simulink model "propulsion"  (R2025b)
settings: Solver=VariableStepAuto  StartTime=0.0  StopTime=10.0  RelTol=1e-3
undefined symbols (not defined in the file or in its folder): DiscIntNeverNeededParam
settings Model: Creator=taeta  LastModifiedBy=taeta

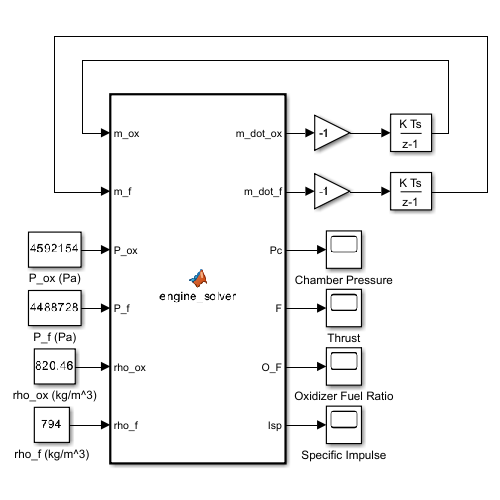
[thumbnail: Simulink's stored preview of the top-level diagram]
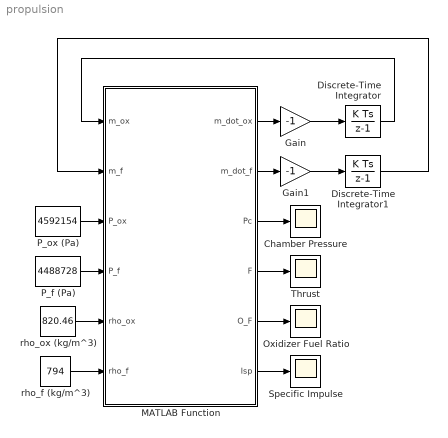
== system propulsion ==
  Chamber Pressure : Scope
      settings: ActiveDisplayYMinimum=-1  ActiveDisplayYMaximum=1
  Discrete-Time Integrator : DiscreteIntegrator  InitialCondition=33.8916  SampleTime=-1  ICPrevOutput=DiscIntNeverNeededParam  ICPrevScaledInput=DiscIntNeverNeededParam
  Discrete-Time Integrator1 : DiscreteIntegrator  InitialCondition=9.678  SampleTime=-1  ICPrevOutput=DiscIntNeverNeededParam  ICPrevScaledInput=DiscIntNeverNeededParam
  Gain : Gain  Gain=-1
  Gain1 : Gain  Gain=-1
  MATLAB Function : MATLAB Function  TreatAsAtomicUnit=on
  Oxidizer Fuel Ratio : Scope
      settings: ActiveDisplayYMinimum=-1  ActiveDisplayYMaximum=1  DataLoggingVariableName=ScopeData2
  P_f (Pa) : Constant  Value=4488728
  P_ox (Pa) : Constant  Value=4592154
  Specific Impulse : Scope
      settings: ActiveDisplayYMinimum=-1  ActiveDisplayYMaximum=1  DataLoggingVariableName=ScopeData3
  Thrust : Scope
      settings: ActiveDisplayYMinimum=-1  ActiveDisplayYMaximum=1
  rho_f (kg/m^3) : Constant  Value=794
  rho_ox (kg/m^3) : Constant  Value=820.46
  wires:
  MATLAB Function/1(m_dot_ox) -> Gain/1
  MATLAB Function/2(m_dot_f) -> Gain1/1
  Discrete-Time Integrator/1 -> MATLAB Function/1(m_ox)
  Discrete-Time Integrator1/1 -> MATLAB Function/2(m_f)
  Gain/1 -> Discrete-Time Integrator/1
  Gain1/1 -> Discrete-Time Integrator1/1
  rho_f (kg/m^3)/1 -> MATLAB Function/6(rho_f)
  rho_ox (kg/m^3)/1 -> MATLAB Function/5(rho_ox)
  P_ox (Pa)/1 -> MATLAB Function/3(P_ox)
  P_f (Pa)/1 -> MATLAB Function/4(P_f)
  MATLAB Function/6(Isp) -> Specific Impulse/1
  MATLAB Function/5(O_F) -> Oxidizer Fuel Ratio/1
  MATLAB Function/4(F) -> Thrust/1
  MATLAB Function/3(Pc) -> Chamber Pressure/1

== matlab function propulsion/MATLAB Function ==
  data: m_ox input; m_dot_ox output; m_f input; P_ox input; P_f input; rho_ox input; rho_f input; m_dot_f output; Pc output; F output; O_F output; Isp output
function [m_dot_ox, m_dot_f, Pc, F, O_F, Isp] = engine_solver(m_ox, m_f, P_ox, P_f, rho_ox, rho_f)

    % output dimensions for simulink (everything equals 0 at first)
    m_dot_ox = 0;
    m_dot_f = 0;
    Pc = 0;
    F = 0;
    O_F = 0;
    Isp = 0;

    % constants
    g0 = 9.81; % m/s^2
    c_star = 2639.4; % m/s
    A_t = 7.85398e-5; % m^2
    A_e = 1.8816e-3; % m^2
    C_f = A_e / A_t; % thrust coefficient

    % initial guesses [m_dot_ox (kg/s); m_dot_f (kg/s); Pc (Pa)]
    x0 = [1.66337; 0.478249; 435.113 * 6894.76];

    % optimization for simulink or else it wont work
    options = optimoptions('fsolve', ...
        'Algorithm', 'levenberg-marquardt', ...
        'Display', 'off', ...
        'FunctionTolerance', 1e-6);

    % solve non-linear residual system
    [x_sol, ~, exitflag] = fsolve(@(x) engine_residuals(x, P_ox, P_f, rho_ox, rho_f, A_t, c_star), x0, options);

    if exitflag <= 0
        x_sol = x0; % so if solver fails to converge it like fixes itself basiaclly
    end

    % gets the solved state values
    m_dot_ox = abs(x_sol(1));
    m_dot_f = abs(x_sol(2));
    Pc = abs(x_sol(3));

    % engine performance outputs
    m_dot_tot = m_dot_ox + m_dot_f;
    F = C_f * Pc * A_t;
    O_F = m_dot_ox / max(m_dot_f, 1e-6);
    Isp = F / (max(m_dot_tot, 1e-6) * g0);
end

function R = engine_residuals(x, P_ox, P_f, rho_ox, rho_f, A_t, c_star)
    m_dot_ox_guess = abs(x(1));
    m_dot_f_guess = abs(x(2));
    Pc_guess = abs(x(3));

    % line losses using oxidizer and fuel constants
    dp_ox = calculate_line_loss_ox(m_dot_ox_guess, rho_ox);
    dp_f = calculate_line_loss_f(m_dot_f_guess, rho_f);

    % residual equations (assuming we want R=0)
    R_ox = P_ox - dp_ox - Pc_guess;
    R_f = P_f - dp_f - Pc_guess;
    R_c = (m_dot_ox_guess + m_dot_f_guess) - (Pc_guess * A_t / c_star);

    R = [R_ox; R_f; R_c];

    % this is so NaN/inf doesnt happen to fsolve
    if any(~isfinite(R))
        R = [1e6; 1e6; 1e6];
    end
end

function dp = calculate_line_loss_ox(m_dot, rho)
    % oxidizer line parameters
    g0 = 9.81;
    rho_safe = max(rho, 1e-3);
    
    f = 0.04; % friction factor
    D = 0.0535088; % pipe diameter (m)
    L = 0.762; % pipe length (m)
    k = 10; % minor loss coefficient
    Cv = 9; % valve flow coefficient
    A_inj = 2.20893e-5; % injector area (m^2)
    dz = 0.9144; % elevation change (m)
    
    % velocity and dynamic pressur
    A_pipe = (pi / 4) * D^2;
    v = m_dot / (rho_safe * A_pipe);
    q = 0.5 * rho_safe * (v^2);

    % individual pressure loss terms
    dp_pipe = f * (L / D) * q; % pipe loss
    dp_k = k * q; % minor loss
    
    % valve loss: i made it so that it converts m_dot to GPM for Cv equation
    SG = rho_safe / 1000; % specific gravity
    Q_gpm = (m_dot / rho_safe) * 15850.32; % m^3/s to GPM
    dp_v = SG * (Q_gpm / Cv)^2 * 6894.76; % converted psi to Pa
    
    dp_inj = 0.5 * (m_dot / A_inj)^2 / rho_safe; % injector loss
    dp_g = rho_safe * g0 * dz; % hydrostatic loss

    % total oxidizer pressure drop (Pa)
    dp = dp_pipe + dp_k + dp_v + dp_inj + dp_g;
end

function dp = calculate_line_loss_f(m_dot, rho)
    % fuel fine parameters
    g0 = 9.81;
    rho_safe = max(rho, 1e-3);
    f = 0.04; % friction factor
    D = 0.01270; % pipe diameter (m)
    L = 0.762; % pipe length (m)
    k = 10; % minor loss coefficient
    Cv = 5.228; % valve flow coefficient
    A_inj = 1.8816e-3; % injector area (m^2)
    dz= 0.9144; % elevation change (m)

    % velocity and dynamics pressue
    A_pipe = (pi / 4) * D^2;
    v = m_dot / (rho_safe * A_pipe);
    q = 0.5 * rho_safe * (v^2);

    % individual pressure loss terms
    dp_pipe = f * (L / D) * q;
    dp_k = k * q;
    
    SG = rho_safe / 1000;
    Q_gpm = (m_dot / rho_safe) * 15850.32;
    dp_v = SG * (Q_gpm / Cv)^2 * 6894.76;
    
    dp_inj = 0.5 * (m_dot / A_inj)^2 / rho_safe;
    dp_g = rho_safe * g0 * dz;

    % total fuel pressure drop (Pa)
    dp = dp_pipe + dp_k + dp_v + dp_inj + dp_g;
end
